simulink model "Model_1"  (R2020b)
settings: Solver=VariableStepAuto  StartTime=0.0  StopTime=10.0  RelTol=1e-3
libraries: simulink_extras x1
settings Model: EnablePacing=on  PacingRate=0.700000  Creator=Akarsh  LastModifiedBy=Akarsh

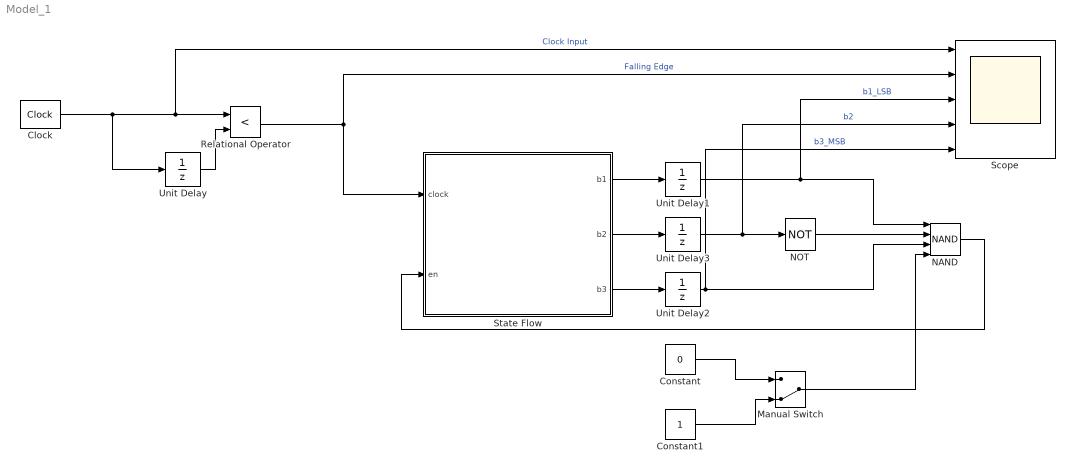
== system Model_1 ==
  Clock : simulink_extras/Flip Flops/Clock  period=1
  Constant : Constant  Value=0
  Constant1 : Constant
  Manual Switch : ManualSwitch  CurrentSetting=0
  NAND : Logic  Operator=NAND  Inputs=4  IconShape=distinctive  AllPortsSameDT=off  OutDataTypeStr=boolean
  NOT : Logic  Operator=NOT  IconShape=distinctive  AllPortsSameDT=off  OutDataTypeStr=boolean
  Relational Operator : RelationalOperator  Operator=<  OutDataTypeStr=boolean  RndMeth=Simplest
  Scope : Scope  NumInputPorts=5
  State Flow : Stateflow chart  TreatAsAtomicUnit=on
  Unit Delay{,1..3} (4 alike) : UnitDelay  SampleTime=-1  HasFrameUpgradeWarning=on
  wires:
  Clock/1 -> Relational Operator/1, Scope/1, Unit Delay/1  "Clock Input"
  Unit Delay/1 -> Relational Operator/2
  Relational Operator/1 -> Scope/2, State Flow/1(clock)  "Falling Edge"
  State Flow/1(b1) -> Unit Delay1/1
  State Flow/2(b2) -> Unit Delay3/1
  State Flow/3(b3) -> Unit Delay2/1
  Unit Delay3/1 -> Scope/4, NOT/1  "b2"
  Unit Delay1/1 -> Scope/3, NAND/1  "b1_LSB"
  NOT/1 -> NAND/2
  Constant/1 -> Manual Switch/1
  Constant1/1 -> Manual Switch/2
  Manual Switch/1 -> NAND/4
  Unit Delay2/1 -> Scope/5, NAND/3  "b3_MSB"
  NAND/1 -> State Flow/2(en)

== stateflow chart Model_1/State Flow ==
  state State_1
    en:b1=0;
    b2=0;
    b3=0;
  state State_2
    en: b1 = 1;
    b2 = 0;
    b3 = 0;
  state State_8
    en: b1 = 1;
    b2 = 0;
    b3 = 0;
  state State_3
    en: b1 = 1;
    b2 = 0;
    b3 = 0;
  state State_7
    en: b1 = 1;
    b2 = 0;
    b3 = 0;
  state State_4
    en: b1 = 1;
    b2 = 0;
    b3 = 0;
  state State_6
    en: b1 = 1;
    b2 = 0;
    b3 = 0;
  state State_5
    en: b1 = 1;
    b2 = 0;
    b3 = 0;
  (default) -> State_1
  State_1 -> State_2 : [clock==1]
  State_8 -> State_1 : [clock==1]
  (junction 19) -> State_1 [order 2] : [en==1]
  State_2 -> State_3 : [clock==1]
  State_7 -> State_8 : [clock==1]
  State_3 -> State_4 : [clock==1]
  State_5 -> (junction 19) : [clock==1]
  (junction 19) -> State_6 [order 1] : [en==0]
  State_6 -> State_7 : [clock==1]
  State_4 -> State_5 : [clock==1]
  data: clock input; en input; b1 output; b2 output; b3 output
